simulink model "Kia_Niro_Powertrain_Model3"  (R2025a)
settings: Solver=ode1  StartTime=0.0  StopTime=inf  FixedStep=0.001  RelTol=1e-3  EnableMultiTasking=on
values from neighbouring files (symbols this model uses):
  B = 0.001    [Torque_maps.m]
  Fz_breakpoints = [2000, 3000, 4000, 5000, 6000]    [slip_controller.m]
  J = 0.00019    [Torque_maps.m]
  Kc_d = 0    [Torque_maps.m]
  Kc_i = 2E3    (= 2000)    [Torque_maps.m]
  Kc_p = 32    [Torque_maps.m]
  Ldq = L1+Lm    (= 0.088)    [Torque_maps.m]
  M = Ke/(sqrt(3)*PP)    [Torque_maps.m]
  Mu_breakpoints = [0.2, 0.4, 0.6, 0.8, 1.0]    [slip_controller.m]
  pedal_bp_negative = -1:0.05:0    [Torque_maps.m]
  pedal_bp_positive = 0:0.05:1    [Torque_maps.m]
  PP = 2    [Torque_maps.m]
  rpm_bp = 0:250:14125    [Torque_maps.m]
  Rs = 32    [Torque_maps.m]
  T2Iconversion = 2/(3*M*PP)    [Torque_maps.m]
  Target_Slip_Table = [ ... (first row only)    [slip_controller.m]
  torque_table_negative = zeros(length(rpm_bp), length(pedal_bp_negative))    [Torque_maps.m]
  torque_table_positive = zeros(length(rpm_bp), length(pedal_bp_positive))    [Torque_maps.m]
  Vdc = 335/2    (= 167.5)    [Torque_maps.m]
undefined symbols (not defined in the file or in its folder): DiscIntNeverNeededParam
libraries: CarMaker4SL x18, slpidlib x4, eeTransforms x2, autolibpmsmexterior x1
(part 4 of 4)

== system Kia_Niro_Powertrain_Model3/CarMaker/IPG Vehicle/PowerTrain/Slip Controller/Braking/Subsystem ==
  Pedal_demand_Trq : Inport
  u : Inport  Port=2
  Reset : Inport  Port=3
  Abs : Abs  SaturateOnIntegerOverflow=off
  Constant1 : Constant  Value=0
  Discrete PID Controller : slpidlib/PID Controller  Controller=PI  Form=Parallel  TimeDomain=Discrete-time  UseExternalTs=off  SampleTime=-1  IntegratorMethod=Forward Euler  FilterMethod=Forward Euler  ControllerParametersSource=internal  P=2000  I=2500  UseKiTs=off  D=10000  UseExternalDerivativeSource=off  N=100  UseFilter=on  TunerSelectOption=Transfer Function Based (PID Tuner App)  InitialConditionSource=internal  InitialConditionForIntegrator=0  InitialConditionForFilter=0  DifferentiatorICPrevScaledInput=0  ExternalReset=level  TrackingMode=off  Kt=1  LimitOutput=on  SatLimitsSource=external  UpperSaturationLimit=inf  LowerSaturationLimit=-inf  LinearizeAsGain=off  AntiWindupMode=back-calculation  Kb=1  LimitIntegrator=off  UpperIntegratorSaturationLimit=inf  LowerIntegratorSaturationLimit=-inf  RndMeth=Nearest  POutMin=[]  POutMax=[]  IOutMin=[]  IOutMax=[]  DOutMin=[]  DOutMax=[]  NOutMin=[]  NOutMax=[]  SumOutMin=[]  SumOutMax=[]  SaturationOutMin=[]  SaturationOutMax=[]  PParamMin=[]  PParamMax=[]  IParamMin=[]  IParamMax=[]  DParamMin=[]  DParamMax=[]  NParamMin=[]  NParamMax=[]  KbParamMin=[]  KbParamMax=[]  KtParamMin=[]  KtParamMax=[]  KbOutMin=[]  KbOutMax=[]  KtOutMin=[]  KtOutMax=[]  IntegratorOutMin=[]  IntegratorOutMax=[]  FilterOutMin=[]  FilterOutMax=[]  SumI1OutMin=[]  SumI1OutMax=[]  SumI2OutMin=[]  SumI2OutMax=[]  SumI3OutMin=[]  SumI3OutMax=[]  SumI4OutMin=[]  SumI4OutMax=[]  SumDOutMin=[]  SumDOutMax=[]  DifferentiatorOutMin=[]  DifferentiatorOutMax=[]  FilterDiffOutCoefMin=[]  FilterDiffOutCoefMax=[]  ReciprocalOutMin=[]  ReciprocalOutMax=[]  SumDenOutMin=[]  SumDenOutMax=[]  SumNumOutMin=[]  SumNumOutMax=[]  DivideOutMin=[]  DivideOutMax=[]  UdiffTsProdOutMin=[]  UdiffTsProdOutMax=[]  NTsProdOutMin=[]  NTsProdOutMax=[]  UintegralTsProdOutMin=[]  UintegralTsProdOutMax=[]  UngainTsProdOutMin=[]  UngainTsProdOutMax=[]  ClampingZeroOutDataTypeStr=Inherit: Inherit via back propagation  ClampingZeroOutMin=[]  ClampingZeroOutMax=[]  FilterDenConstantOutDataTypeStr=Inherit: Inherit via back propagation  FilterDenConstantOutMin=[]  FilterDenConstantOutMax=[]  PCopyOutDataTypeStr=Inherit: Inherit via back propagation  PCopyOutMin=[]  PCopyOutMax=[]  NCopyOutDataTypeStr=Inherit: Inherit via back propagation  NCopyOutMin=[]  NCopyOutMax=[]  IntegratorContinuousStateAttributes=''  IntegratorStateMustResolveToSignalObject=off  IntegratorRTWStateStorageClass=Auto  FilterContinuousStateAttributes=''  FilterStateMustResolveToSignalObject=off  FilterRTWStateStorageClass=Auto  ParallelPVariant=InternalParameters  IdealPVariant=Disabled  IVariant=InternalParameters  DVariant=Disabled  IntegratorVariant=Discrete  SatVariant=External  AWVariant=BackCalculation  PCopyVariant=Disabled  TRVariant=Disabled  FdbkBlocksVariant=Forward  IdealPFdbkVariant=Disabled  SatFdbkVariant=Disabled  DerivativeFilterVariant=Disabled  NVariant=Disabled  NCopyVariant=Disabled_SignalSpec  FilterICVariant=Disabled  IntegratorICVariant=InternalICs  ExternalResetVariant=ExternalReset  TRSumVariant=Passthrough  SumFdbkVariant=Disabled  SumVariant=Sum_PI  TsampFilterVariant=InternalTs  TsampNgainVariant=Passthrough  TsampIntegralVariant=Disabled_SignalSpec  ExternalSaturationOutDataTypeStr=Inherit: Same as second input  DerivativeSourceVariant=Disabled  PreIntVariant=InternalPreInt
      settings: LibrarySourceBlock=simulink/Discrete/Discrete PID Controller
  Correction Trq : Outport
  wires:
  Constant1/1 -> Discrete PID Controller/4
  Discrete PID Controller/1 -> Correction Trq/1  "Correction Trq"
  Pedal_demand_Trq/1 -> Abs/1
  u/1 -> Discrete PID Controller/1
  Abs/1 -> Discrete PID Controller/3
  Reset/1 -> Discrete PID Controller/2

== system Kia_Niro_Powertrain_Model3/CarMaker/IPG Vehicle/PowerTrain/User RearDriven PowerTrain/Motor Model/Cross Coupling Removal ==
  control_Vd : Inport
  Id : Inport  Port=2
  Iq : Inport  Port=3
  control_Vq : Inport  Port=4
  rotor_electrical_speed : Inport  Port=5
  MATLAB Function : MATLAB Function  TreatAsAtomicUnit=on
  target_Vd : Outport
  target_Vq : Outport  Port=2
  wires:
  Iq/1 -> MATLAB Function/2(Iq)
  rotor_electrical_speed/1 -> MATLAB Function/5(rotor_electrical_speed)
  control_Vd/1 -> MATLAB Function/3(control_Vd)
  Id/1 -> MATLAB Function/1(Id)
  MATLAB Function/1(target_Vd) -> target_Vd/1
  MATLAB Function/2(target_Vq) -> target_Vq/1
  control_Vq/1 -> MATLAB Function/4(control_Vq)

== system Kia_Niro_Powertrain_Model3/CarMaker/IPG Vehicle/PowerTrain/User RearDriven PowerTrain/Motor Model/Current Reference Generator ==
  In1 : Inport
  Constant1 : Constant  Value=0
  Gain4 : Gain  Gain=T2Iconversion
  target_Id : Outport
  target_Iq : Outport  Port=2
  wires:
  In1/1 -> Gain4/1
  Gain4/1 -> target_Iq/1  "target_Iq"
  Constant1/1 -> target_Id/1  "target_Id"

== system Kia_Niro_Powertrain_Model3/CarMaker/IPG Vehicle/PowerTrain/User RearDriven PowerTrain/Subsystem1/COLOUMB COUNTING1 ==
  note: total capacity (mAh)
  note: A . sec
  note: mAh
  note: A . sec
  note: total capacity (mAh)
  note: mAh
  current real : Inport
  current coloumb : Inport  Port=2
  (As) to (mAh) : Gain  Gain=1000/3600
  (As) to (mAh)1 : Gain  Gain=1000/3600
  Battery total capacity (mAh) : Constant  Value=4800
  Battery total capacity (mAh)1 : Constant  Value=4800
  Discrete-Time Integrator1 : DiscreteIntegrator  SampleTime=0.01  ICPrevOutput=DiscIntNeverNeededParam  ICPrevScaledInput=DiscIntNeverNeededParam
  Integrator : Integrator
  MATLAB Function : MATLAB Function  TreatAsAtomicUnit=on
  MATLAB Function1 : MATLAB Function  TreatAsAtomicUnit=on
  Relational Operator : RelationalOperator  Operator=<=  OutDataTypeStr=boolean  InputSameDT=off
  Relational Operator1 : RelationalOperator  Operator=<=  OutDataTypeStr=boolean  InputSameDT=off
  Stop Simulation : Stop
  Stop Simulation1 : Stop
  initial SOC (%) : Constant  Value=80
  initial SOC (%)1 : Constant  Value=80
  zero1 : Constant  Value=0
  zero2 : Constant  Value=0
  S_real : Outport
  S_col : Outport  Port=2
  wires:
  MATLAB Function/1(SoC) -> S_col/1, Relational Operator/1
  (As) to (mAh)/1 -> MATLAB Function/3(I)
  current coloumb/1 -> Discrete-Time Integrator1/1
  Relational Operator/1 -> Stop Simulation/1
  Battery total capacity (mAh)/1 -> MATLAB Function/1(Ct)
  initial SOC (%)/1 -> MATLAB Function/2(SOC_init)
  zero2/1 -> Relational Operator/2
  zero1/1 -> Relational Operator1/2
  Relational Operator1/1 -> Stop Simulation1/1
  initial SOC (%)1/1 -> MATLAB Function1/2(SOC_init)
  current real/1 -> Integrator/1
  Battery total capacity (mAh)1/1 -> MATLAB Function1/1(Ct)
  (As) to (mAh)1/1 -> MATLAB Function1/3(I)
  MATLAB Function1/1(SoC) -> S_real/1, Relational Operator1/1
  Integrator/1 -> (As) to (mAh)1/1
  Discrete-Time Integrator1/1 -> (As) to (mAh)/1

== system Kia_Niro_Powertrain_Model3/CarMaker/IPG Vehicle/PowerTrain/User RearDriven PowerTrain/Subsystem1/Parameter updating1 ==
  SoC : Inport
  Gain : Gain
  Poly_R1 : Polyval  Coefs=[1.466124009149211e-08,-3.016114306306107e-06,2.169854530489312e-04,-0.006504304448579,0.091010234125850]
  Ro Lookup Table : Lookup_n-D  NumberOfTableDimensions=1  BreakpointsForDimension1="[0\t5\t7\t9\t11\t13\t15\t17\t19\t21\t23\t25\t27\t29\t31\t33\t35\t37\t39\t41\t43\t45\t47\t49\t51\t53\t55\t57\t59\t61\t63\t65\t67\t69\t71\t73\t75\t77\t79\t81\t83\t85\t87\t89\t91\t93\t95\t97\t100]"  Table="[0.140000000000000\t0.110000000000000\t0.110000000000000\t0.100000000000000\t0.0900000000000000\t0.0900000000000000\t0.0800000000000000\t0.0800000000000000\t0.0700000000000000\t0.0700000000000000\t0.0700000000000000\t0.0700000000000000\t0.0700000000000000\t0.0700000000000000\t0.0700000000000000\t0.0700000000000000\t0.0700000000000000\t0.0600000000000000\t0.0700000000000000\t0.0600000000000000\t0.0600000000000000\t0.0700000000000000\t0.0600000000000000\t0.0700000000000000\t0.0610000000000000\t0.0620000000000000\t0.0630000000000000\t0.0640000000000000\t0.0660000000000000\t0.0650000000000000\t0.0670000000000000\t0.0610000000000000\t0.0610000000000000\t0.0620000000000000\t0.0630000000000000\t0.0620000000000000\t0.0640000000000000\t0.0640000000000000\t0.0650000000000000\t0.0640000000000000\t0.0680000000000000\t0.0710000000000000\t0.0710000000000000\t0.0720000000000000\t0.0740000000000000\t0.0740000000000000\t0.0740000000000000\t0.0750000000000000\t0.0770000000000000]"  InternalRulePriority=Speed  RndMeth=Simplest
  Ro Lookup Table1 : Lookup_n-D  NumberOfTableDimensions=1  BreakpointsForDimension1=[0 5 7 9 11 13 15 17 19 21 23 25 27 29 31 33 35 37 39 41 43 45 47 49 51 53 55 57 59 61 63 65 67 69 71 73 75 77 79 81 83 85 87 89 91 93 95 97 100]  Table=[-0.59999999999999998 -0.42857142857142899 -0.25 -0.5 -0.25 -0.25 -0.25 -0.25 -0.25 0 0 0 0 0 0 0 -0.25 0 0 -0.25 0.25 0 0 0.025000000000000001 -0.20000000000000001 0.050000000000000003 0.050000000000000003 0.074999999999999997 0.025000000000000001 0.025000000000000001 -0.10000000000000001 -0.14999999999999999 0.025000000000000001 0.050000000000000003 0 0.025000000000000001 0.050000000000000003 0.025000000000000001 0 0.074999999999999997 0.17499999999999999 0.074999999999999997 0.025000000000000001 0.074999999999999997 0.050000000000000003 0 0.025000000000000001 0.059999999999999998 0.066666666666666999]  InternalRulePriority=Speed  RndMeth=Simplest
  Voc Lookup Table : Lookup_n-D  NumberOfTableDimensions=1  BreakpointsForDimension1="[0\t5\t7\t9\t11\t13\t15\t17\t19\t21\t23\t25\t27\t29\t31\t33\t35\t37\t39\t41\t43\t45\t47\t49\t51\t53\t55\t57\t59\t61\t63\t65\t67\t69\t71\t73\t75\t77\t79\t81\t83\t85\t87\t89\t91\t93\t95\t97\t100]"  Table="[7.01000000000000\t7.09000000000000\t7.16000000000000\t7.20000000000000\t7.29000000000000\t7.34000000000000\t7.38000000000000\t7.41000000000000\t7.44000000000000\t7.47000000000000\t7.49000000000000\t7.52000000000000\t7.54000000000000\t7.56000000000000\t7.58000000000000\t7.60000000000000\t7.61000000000000\t7.63000000000000\t7.64000000000000\t7.65000000000000\t7.66000000000000\t7.67000000000000\t7.68000000000000\t7.69000000000000\t7.69800000000000\t7.70200000000000\t7.71100000000000\t7.71400000000000\t7.72000000000000\t7.72800000000000\t7.73500000000000\t7.74000000000000\t7.74500000000000\t7.75400000000000\t7.75800000000000\t7.76100000000000\t7.76800000000000\t7.77500000000000\t7.77800000000000\t7.79000000000000\t7.80900000000000\t7.85100000000000\t7.87000000000000\t7.92300000000000\t7.98100000000000\t8.05500000000000\t8.15200000000000\t8.26600000000000\t8.44300000000000]"  InternalRulePriority=Speed  RndMeth=Simplest
  Voc Lookup Table1 : Lookup_n-D  NumberOfTableDimensions=1  BreakpointsForDimension1=[0 5 7 9 11 13 15 17 19 21 23 25 27 29 31 33 35 37 39 41 43 45 47 49 51 53 55 57 59 61 63 65 67 69 71 73 75 77 79 81 83 85 87 89 91 93 95 97 100]  Table=[1.600000000000001 2.142857142857148 2.750000000000008 3.249999999999998 3.499999999999991 2.249999999999997 1.750000000000007 1.500000000000012 1.499999999999991 1.249999999999995 1.249999999999995 1.249999999999995 1.000000000000001 1.000000000000001 1 0.750000000000007 0.750000000000007 0.749999999999983 0.500000000000012 0.500000000000012 0.499999999999989 0.49999999999999 0.500000000000012 0.450000000000017 0.299999999999989 0.324999999999997 0.300000000000012 0.224999999999987 0.349999999999983 0.375000000000014 0.300000000000011 0.249999999999994 0.349999999999984 0.324999999999998 0.175000000000014 0.249999999999994 0.350000000000006 0.249999999999994 0.374999999999992 0.775000000000016 1.525000000000001 1.524999999999997 1.8 2.774999999999991 3.299999999999989 4.274999999999992 5.275000000000017 5.820000000000002 5.899999999999982]  InternalRulePriority=Speed  RndMeth=Simplest
  poly_C1 : Polyval  Coefs=[-6.954272499766545e-05,0.013572818088594,-0.971124742038101,33.500516588178876,92.374565325126170]
  Voc : Outport
  Ro : Outport  Port=2
  R1 : Outport  Port=3
  C1 : Outport  Port=4
  dVoc : Outport  Port=5
  dR0 : Outport  Port=6
  wires:
  SoC/1 -> Ro Lookup Table1/1, poly_C1/1, Poly_R1/1, Voc Lookup Table1/1, Voc Lookup Table/1, Ro Lookup Table/1
  Voc Lookup Table/1 -> Voc/1
  Ro Lookup Table/1 -> Ro/1
  Poly_R1/1 -> R1/1
  poly_C1/1 -> C1/1
  Voc Lookup Table1/1 -> Gain/1
  Gain/1 -> dVoc/1
  Ro Lookup Table1/1 -> dR0/1

== system Kia_Niro_Powertrain_Model3/CarMaker/IPG Vehicle/PowerTrain/User RearDriven PowerTrain/Subsystem1/RC network subsystem1 ==
  note: D(V1)
  note: V1
  current (A) : Inport
  R1 : Inport  Port=2
  " C1" : Inport  Port=3
  Discrete-Time Integrator1 : DiscreteIntegrator  SampleTime=-1  ICPrevOutput=DiscIntNeverNeededParam  ICPrevScaledInput=DiscIntNeverNeededParam
  MATLAB Function : MATLAB Function  TreatAsAtomicUnit=on
  V1 : Outport
  wires:
  MATLAB Function/1(y) -> Discrete-Time Integrator1/1
  Discrete-Time Integrator1/1 -> MATLAB Function/4(V1), V1/1
  current (A)/1 -> MATLAB Function/1(I)
  R1/1 -> MATLAB Function/2(R1)
  " C1"/1 -> MATLAB Function/3(C1)

== matlab function Kia_Niro_Powertrain_Model3/CarMaker/IPG Vehicle/PowerTrain/User RearDriven PowerTrain/Motor Model/Cross Coupling Removal/MATLAB Function ==
  data: target_Vd output; target_Vq output; Id input; Iq input; control_Vd input; control_Vq input; rotor_electrical_speed input; Ldq parameter; Rs parameter; M parameter; PP parameter; Vdc parameter
function [target_Vd,target_Vq] = fcn(Id,Iq,control_Vd,control_Vq,rotor_electrical_speed, Ldq, Rs, M, PP, Vdc)
% We are using complex variables to simplify the vectorial operation -
% particlarly the time derivative
Idq = Id + i*Iq;
lambda = Ldq*Idq + M;
control_Vdq = control_Vd + i*control_Vq;
% For a vector lambda rotating with speed rotor_electrical_speed, the time
% derivative is i*rotor_electrical_speed*lambda
target_Vdq = control_Vdq + i*rotor_electrical_speed*lambda;
target_Vd = real(target_Vdq);
target_Vq = imag(target_Vdq);
end

== matlab function Kia_Niro_Powertrain_Model3/CarMaker/IPG Vehicle/PowerTrain/User RearDriven PowerTrain/Subsystem1/COLOUMB COUNTING1/MATLAB Function ==
  data: Ct input; SoC output; SOC_init input; I input
function SoC = fcn(Ct,SOC_init,I)

% Ct : Battery total capacity (mAh)
% SOC_init : Initial SoC (%)
% I : Cumulative Current (used capacity in mAh)
% y : SoC

 SoC = SOC_init - 100*(I/Ct) ;

end

== matlab function Kia_Niro_Powertrain_Model3/CarMaker/IPG Vehicle/PowerTrain/User RearDriven PowerTrain/Subsystem1/COLOUMB COUNTING1/MATLAB Function1 ==
  data: Ct input; SoC output; SOC_init input; I input
function SoC = fcn(Ct,SOC_init,I)

% Ct : Battery total capacity (mAh)
% SOC_init : Initial SoC (%)
% I : Cumulative Current (used capacity in mAh)
% y : SoC

 SoC = SOC_init - 100*(I/Ct) ;

end

== matlab function Kia_Niro_Powertrain_Model3/CarMaker/IPG Vehicle/PowerTrain/User RearDriven PowerTrain/Subsystem1/EKF1 ==
  settings: updateMethod=DISCRETE
  data: I input; soc_hat output; UL_meas input; Uoc input; R0 input; R1 input; C1 input; dUoc_dSoc input; reset input; u1_hat output; ul_hat output; innov output; K_out output; P_out output; dR0 input
function [soc_hat, u1_hat, ul_hat, innov, K_out, P_out] = soc_ekf_paper_1rc(I, UL_meas, Uoc, R0, R1, C1, dUoc_dSoc, reset,dR0)

    persistent x_hat P initialized


    Dt  = 0.01;         
    Q0  = 3600 * 4.8;   
    
    Qekf = [1e-8, 0;
            0,    1e-8];

    Rekf = 1e-2;


    if isempty(initialized) || reset
        x_hat = [0.8;
                 0.0];

        P = [1e-6, 0;
             0,    1e-6];

        initialized = true;
    end

    SOC_k = x_hat(1);
    U1_k  = x_hat(2);
    SOC_k = min(max(SOC_k, 0.0), 1.0);


    tau1 = R1 * C1;
    a1 = exp(-Dt / tau1);

    A = [1,  0;
         0, a1];

    B = [-Dt / Q0;
         R1 * (1 - exp(-(Dt/tau1)))];

    % =========================================================
    % (1) STATE PREDICTION
    % X(k|k-1) = A X(k-1|k-1) + B U(k-1)
    % =========================================================
    x_pred = A * x_hat + B * I;

    

    
    % (2) COVARIANCE PREDICTION
    % P(k|k-1) = A P(k-1) A' + Q
    
    P_pred = A * P * A.' + Qekf;

    
    % (3) MEASUREMENT JACOBIAN
    % C(k) = dg/dx = [dUoc/dSOC, 1]
    
    C = [dUoc_dSoc-dR0*I, -1];

    
    % PREDICTED OUTPUT
    % UL(k) = Uoc(SOC(k)) + I(k)R0 + U1(k)
    
    ul_hat = Uoc - R0 * I - x_pred(2);

    
    % (4) KALMAN GAIN
    % K = P C' (C P C' + R)^(-1)
   
    S = C * P_pred * C.' + Rekf;
  

    K = (P_pred * C.') / S;

    
    % (5) STATE UPDATE
    % X(k|k) = X(k|k-1) + K [ Z(k) - g(X(k),U(k)) ]
    
    innov = UL_meas - ul_hat;

    x_hat = x_pred + K * innov;
    

    
    % (6) COVARIANCE UPDATE
    % P(k|k) = [I - K C] P(k|k-1)
  
    I2 = eye(2);
    %P = (I2 - K*C) * P_pred * (I2 - K*C).' + K*Rekf*K.';
    P = (I2 - K*C) * P_pred ;

    % Outputs
    soc_hat = x_hat(1);
    u1_hat  = x_hat(2);
    K_out   = K;
    P_out   = P;
end

== matlab function Kia_Niro_Powertrain_Model3/CarMaker/IPG Vehicle/PowerTrain/User RearDriven PowerTrain/Subsystem1/RC network subsystem1/MATLAB Function ==
  data: I input; y output; R1 input; C1 input; V1 input
function y = fcn(I,R1,C1,V1)

y = -V1/(R1*C1)+I/C1;
